simulink model "Simple_Vehicle_Model"  (R2019a)
settings: Solver=VariableStepAuto  StartTime=0.0  StopTime=1220  RelTol=1e-3
libraries: qss_tb_library x2, simulink x2
settings Model: Creator=Sai_Mj  LastModifiedBy=Sai_Mj

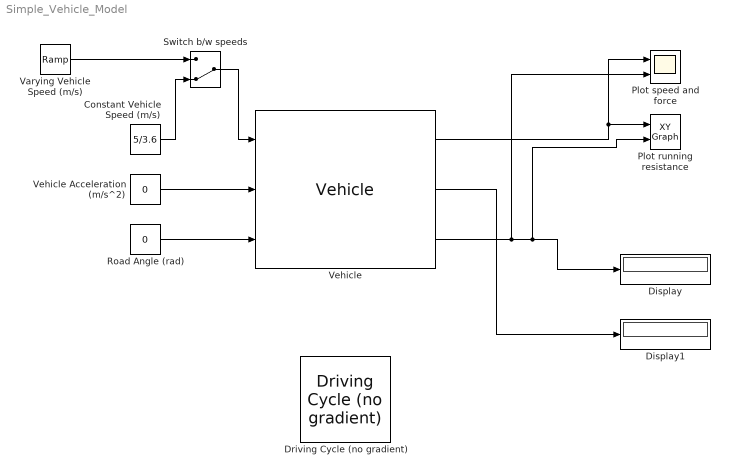
== system Simple_Vehicle_Model ==
  Constant Vehicle Speed (m/s) : Constant  Value=5/3.6
  "Display " : Display
  "Display1 " : Display
  "Driving Cycle (no gradient) " : qss_tb_library/Driving Cycle/Driving Cycle (no gradient)  Tag=cycle  cyclename1=NEDC  stepsize=1  autostop=on
  Plot running resistance : simulink/Sinks/XY Graph  xmin=0  xmax=200/3.6  ymin=0  ymax=2000  st=-1
  Plot speed and force : Scope  NumInputPorts=2
  Road Angle (rad) : Constant  Value=0
  Switch b/w speeds : ManualSwitch  CurrentSetting=0
  "Varying Vehicle Speed (m/s) " : simulink/Sources/Ramp  slope=200/3.6/10  start=0  InitialOutput=0
  "Vehicle " : qss_tb_library/Vehicle/Vehicle  Tag=vehicle  m_f=1700  A_f=2.5  cw=0.31  mu=0.012  k_inertia=5
  Vehicle Acceleration (m/s^2) : Constant  Value=0
  wires:
  "Vehicle "/3 -> Plot speed and force/2, Plot running resistance/2, "Display "/1
  Vehicle Acceleration (m/s^2)/1 -> "Vehicle "/2
  Road Angle (rad)/1 -> "Vehicle "/3
  "Vehicle "/1 -> Plot speed and force/1, Plot running resistance/1
  "Vehicle "/2 -> "Display1 "/1
  Constant Vehicle Speed (m/s)/1 -> Switch b/w speeds/2
  "Varying Vehicle Speed (m/s) "/1 -> Switch b/w speeds/1
  Switch b/w speeds/1 -> "Vehicle "/1
